simulink model "x29sim"  (R2019b)
settings: Solver=VariableStepAuto  StartTime=0.0  StopTime=100  RelTol=1e-3
values from neighbouring files (symbols this model uses):
  A = [0 0       0        1 ... (first row only)    [fbexample.m]    (also in new_dynamics.m = [A_longitude_hi(2,2), A_longitude_hi(2,4), A_longitude_hi(2,; setup_sim.m = A_hi; x29soln.m = [  -0.1645   0.0603 -0.9982 0.0442)
  B = [       0 ... (first row only)    [fbexample.m]    (also in new_dynamics.m = [A_longitude_hi(2, end), A_longitude_hi(4, end), A_longitude; setup_sim.m = B_hi; x29soln.m = [-0.0006  0.0007)
  C = eye(4)    [fbexample.m]    (also in new_dynamics.m = eye(3); second_week.m = pid(-2.29,-1.15); setup_sim.m = eye(18); x29soln.m)
  D = 0    [fbexample.m]    (also in new_dynamics.m = zeros(3,1); setup_sim.m = zeros(18,4); x29soln.m = zeros(4,2))
  d2r = pi/180    (= 0.0174532925199)    [x29soln.m]
  K = place(A,B,[p1,p2,p3,p4])    [fbexample.m]    (also in new_dynamics.m = lqr(A_aug, B_aug, Q, R); x29soln.m = lqr(A_aug, B_aug, Q, R,[]))
  r2d = 180/pi    (= 57.2957795131)    [x29soln.m]
settings Model: Creator=wagneda1  LastModifiedBy=asmialek
settings DataIOCC: ReturnWorkspaceOutputs=off
settings DebuggingCC: ArithmeticOperatorsInVariantConditions=warning
settings SFSimCC: SimUseLocalCustomCode=off  CustomCodeUndefinedFunction=UseInterfaceOnly
settings RTWCC: RTWUseLocalCustomCode=off
settings CodeAppCC: StateflowObjectComments=on

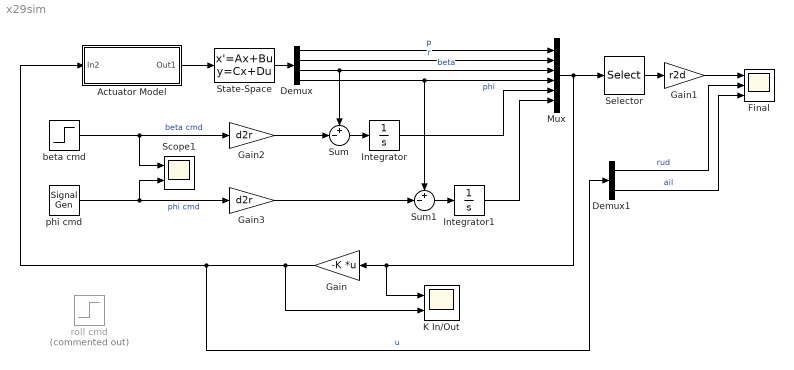
== system x29sim ==
  Actuator Model : Subsystem
  Demux : Demux
  Demux1 : Demux  Outputs=2
  Final : Scope  NumInputPorts=3
  Gain : Gain  Gain=-K  Multiplication=Matrix(K*u)
  Gain1 : Gain  Gain=r2d
  Gain2 : Gain  Gain=d2r
  Gain3 : Gain  Gain=d2r
  Integrator : Integrator
  Integrator1 : Integrator
  K In/Out : Scope  NumInputPorts=2
  Mux : Mux  Inputs=6
  Scope1 : Scope  NumInputPorts=2
  Selector : Selector  InputPortWidth=6  IndexOptions=Index vector (dialog)  Indices=[3 4]  OutputSizes=1
  State-Space : StateSpace  A=A  B=B  C=C  D=D  InitialCondition=0
  Sum : Sum  Inputs=+-|
  Sum1 : Sum  Inputs=+-|
  beta cmd : Step  After=0  SampleTime=0  ZeroCross=off
  phi cmd : SignalGenerator  WaveForm=square  Amplitude=40  Frequency=0.1  Units=rad/sec
  roll cmd : Step  Commented=on  After=-10  SampleTime=0
  wires:
  State-Space/1 -> Demux/1
  Demux/1 -> Mux/1  "p"
  Demux/2 -> Mux/2  "r"
  Demux/3 -> Sum/1, Mux/3  "beta"
  Demux/4 -> Sum1/1, Mux/4  "phi"
  Sum/1 -> Integrator/1
  Sum1/1 -> Integrator1/1
  Integrator/1 -> Mux/5
  Integrator1/1 -> Mux/6
  Mux/1 -> Selector/1, K In/Out/1, Gain/1
  Gain/1 -> K In/Out/2, Actuator Model/1(In2), Demux1/1  "u"
  beta cmd/1 -> Scope1/1, Gain2/1  "beta cmd"
  Demux1/1 -> Final/2  "rud"
  Demux1/2 -> Final/3  "ail"
  Selector/1 -> Gain1/1
  Gain1/1 -> Final/1
  Gain2/1 -> Sum/2
  phi cmd/1 -> Scope1/2, Gain3/1  "phi cmd"
  Gain3/1 -> Sum1/2
  Actuator Model/1(Out1) -> State-Space/1

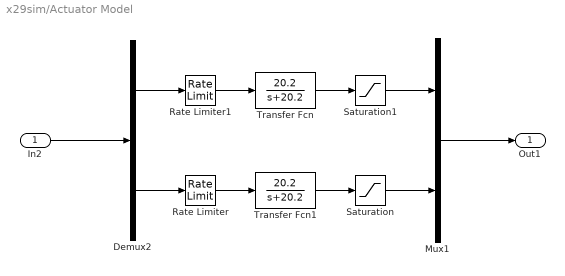
== system x29sim/Actuator Model ==
  In2 : Inport
  Demux2 : Demux  Outputs=2
  Mux1 : Mux  Inputs=2
  Rate Limiter : RateLimiter  RisingSlewLimit=60  FallingSlewLimit=-60  SampleTimeMode=inherited
  Rate Limiter1 : RateLimiter  RisingSlewLimit=60  FallingSlewLimit=-60  SampleTimeMode=inherited
  Saturation : Saturate  UpperLimit=25  LowerLimit=-25
  Saturation1 : Saturate  UpperLimit=25  LowerLimit=-25
  Transfer Fcn : TransferFcn  Numerator=[20.2]  Denominator=[1 20.2]
  Transfer Fcn1 : TransferFcn  Numerator=[20.2]  Denominator=[1 20.2]
  Out1 : Outport
  wires:
  Mux1/1 -> Out1/1
  In2/1 -> Demux2/1
  Transfer Fcn1/1 -> Saturation/1
  Saturation/1 -> Mux1/2
  Transfer Fcn/1 -> Saturation1/1
  Saturation1/1 -> Mux1/1
  Rate Limiter/1 -> Transfer Fcn1/1
  Demux2/2 -> Rate Limiter/1
  Rate Limiter1/1 -> Transfer Fcn/1
  Demux2/1 -> Rate Limiter1/1
